simulink model "Complete_ballsegway_model"  (R2024b)
settings: Solver=VariableStepAuto  StartTime=0.0  StopTime=100  RelTol=1e-3
settings Model: Creator=sumit  LastModifiedBy=sumit

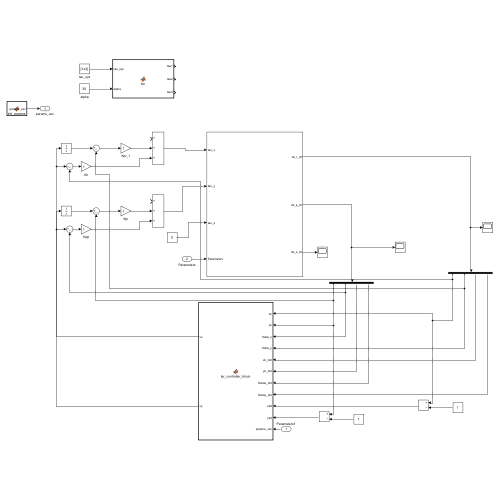
[thumbnail: Simulink's stored preview of the top-level diagram]
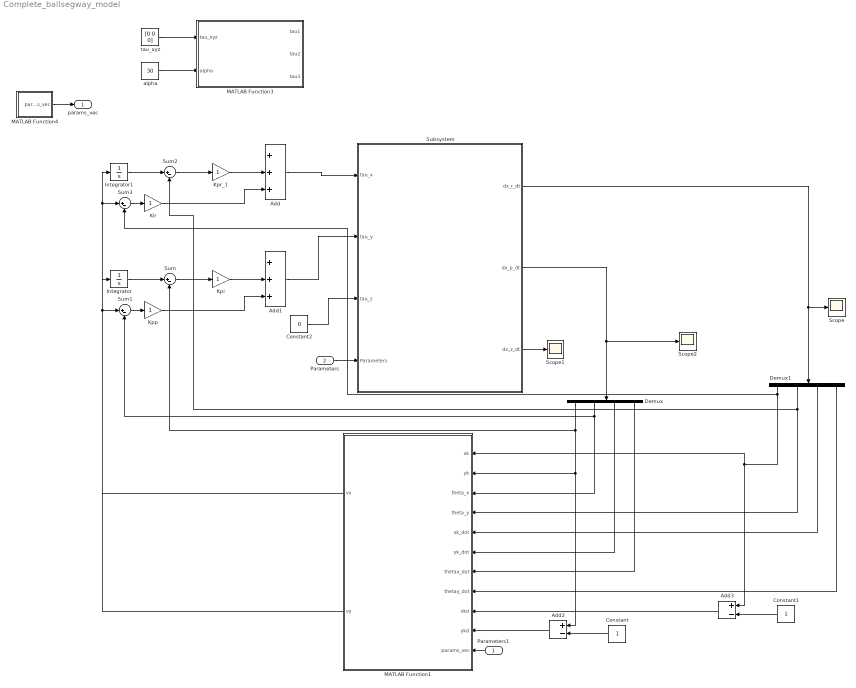
== system Complete_ballsegway_model ==
  Parameters1 : Inport
  Parameters : Inport  Port=2
  Add : Sum  Inputs=+++
  Add1 : Sum  Inputs=+++
  Add2 : Sum  Inputs=+-
  Add3 : Sum  Inputs=+-
  Constant : Constant
  Constant1 : Constant
  Constant2 : Constant  Value=0
  Demux : Demux
  Demux1 : Demux
  Integrator : Integrator
  Integrator1 : Integrator
  Kir : Gain
  Kpi : Gain
  Kpp : Gain
  Kpr_1 : Gain
  MATLAB Function1 : MATLAB Function  TreatAsAtomicUnit=on
  MATLAB Function3 : MATLAB Function  TreatAsAtomicUnit=on
  MATLAB Function4 : MATLAB Function  TreatAsAtomicUnit=on
  Scope : Scope
  Scope1 : Scope
  Scope2 : Scope
  Subsystem : Subsystem
  Sum{,1..3} (4 alike) : Sum  Inputs=|+-
  alpha : Constant  Value=30
  tau_xyz : Constant  Value=[0 0 0]
  params_vec : Outport
  wires:
  alpha/1 -> MATLAB Function3/2(alpha)
  tau_xyz/1 -> MATLAB Function3/1(tau_xyz)
  Subsystem/2(dx_p_dt) -> Demux/1, Scope2/1
  Subsystem/3(dx_z_dt) -> Scope1/1
  Add/1 -> Subsystem/1(tau_x)
  Add1/1 -> Subsystem/2(tau_y)
  Demux/1 -> Sum/2, Add2/1, MATLAB Function1/2(yk)
  Constant/1 -> Add2/2
  Kpi/1 -> Add1/2
  Sum/1 -> Kpi/1
  Integrator/1 -> Sum/1
  Add2/1 -> MATLAB Function1/10(ykd)
  Sum1/1 -> Kpp/1
  Kpp/1 -> Add1/3
  Demux/2 -> Sum1/2, MATLAB Function1/3(theta_x)
  Subsystem/1(dx_r_dt) -> Demux1/1, Scope/1
  MATLAB Function4/1(params_vec) -> params_vec/1
  Parameters/1 -> Subsystem/4(Parameters)
  MATLAB Function1/2(vy) -> Sum1/1, Integrator/1
  Demux/3 -> MATLAB Function1/6(yk_dot)
  Demux/4 -> MATLAB Function1/7(thetax_dot)
  Parameters1/1 -> MATLAB Function1/11(params_vec)
  Demux1/3 -> MATLAB Function1/5(xk_dot)
  Demux1/4 -> MATLAB Function1/8(thetay_dot)
  Constant1/1 -> Add3/2
  Add3/1 -> MATLAB Function1/9(xkd)
  Sum2/1 -> Kpr_1/1
  Kpr_1/1 -> Add/2
  Demux1/2 -> Sum2/2, MATLAB Function1/4(theta_y)
  Demux1/1 -> Sum3/2, Add3/1, MATLAB Function1/1(xk)
  Sum3/1 -> Kir/1
  MATLAB Function1/1(vx) -> Sum3/1, Integrator1/1
  Integrator1/1 -> Sum2/1
  Kir/1 -> Add/3
  Constant2/1 -> Subsystem/3(tau_z)

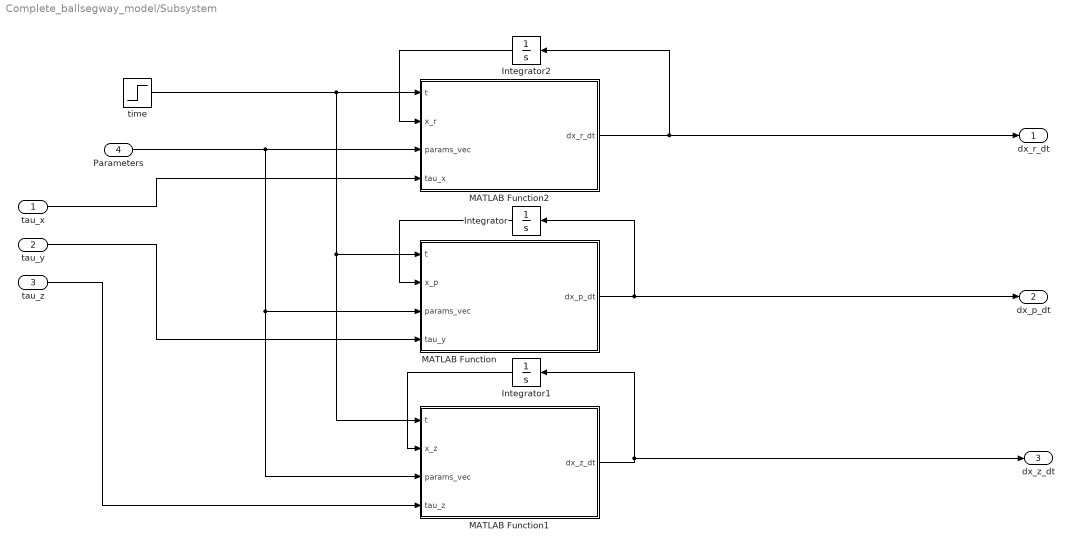
== system Complete_ballsegway_model/Subsystem ==
  tau_x : Inport
  tau_y : Inport  Port=2
  tau_z : Inport  Port=3
  Parameters : Inport  Port=4
  Integrator : Integrator  InitialCondition=[0; 0; 0; 0]
  Integrator1 : Integrator  InitialCondition=[0 ;0]
  Integrator2 : Integrator  InitialCondition=[0; 0; 0; 0]
  MATLAB Function : MATLAB Function  TreatAsAtomicUnit=on
  MATLAB Function1 : MATLAB Function  TreatAsAtomicUnit=on
  MATLAB Function2 : MATLAB Function  TreatAsAtomicUnit=on
  time : Step  After=10  SampleTime=0
  dx_r_dt : Outport
  dx_p_dt : Outport  Port=2
  dx_z_dt : Outport  Port=3
  wires:
  time/1 -> MATLAB Function1/1(t), MATLAB Function/1(t), MATLAB Function2/1(t)
  Integrator1/1 -> MATLAB Function1/2(x_z)
  Parameters/1 -> MATLAB Function/3(params_vec), MATLAB Function1/3(params_vec), MATLAB Function2/3(params_vec)
  Integrator2/1 -> MATLAB Function2/2(x_r)
  MATLAB Function1/1(dx_z_dt) -> Integrator1/1, dx_z_dt/1
  tau_z/1 -> MATLAB Function1/4(tau_z)
  Integrator/1 -> MATLAB Function/2(x_p)
  tau_y/1 -> MATLAB Function/4(tau_y)
  tau_x/1 -> MATLAB Function2/4(tau_x)
  MATLAB Function/1(dx_p_dt) -> Integrator/1, dx_p_dt/1
  MATLAB Function2/1(dx_r_dt) -> dx_r_dt/1, Integrator2/1

== matlab function Complete_ballsegway_model/Subsystem/MATLAB Function1 ==
  data: t input; dx_z_dt output; x_z input; params_vec input; tau_z input
function dx_z_dt = yaw_dynamics(t, x_z, params_vec, tau_z)
% yaw_dynamics.m
%
% 1-DOF yaw dynamic model for Ball Segway.
%
% State x_z = [theta_z ; theta_z_dot]
% params_vec = 20×1 numeric parameter vector (from init_params)
% Output dx_z_dt = state derivative (2×1)

%% ---------------------------------------------------------
% Unpack Parameters From Vector
%% ---------------------------------------------------------

mk  = params_vec(1);     %#ok<NASGU> (not used)
Ik  = params_vec(2);
ma  = params_vec(3);     %#ok<NASGU>
Ix  = params_vec(4);     %#ok<NASGU>
Iy  = params_vec(5);
Iz  = params_vec(6);
l   = params_vec(7);     %#ok<NASGU>
alpha_rad = params_vec(8);
rk  = params_vec(9);
rw  = params_vec(10);
bx  = params_vec(11);    %#ok<NASGU>
dx  = params_vec(12);    %#ok<NASGU>
by  = params_vec(13);    %#ok<NASGU>
dy  = params_vec(14);    %#ok<NASGU>
bry = params_vec(15);    %#ok<NASGU>
dry = params_vec(16);    %#ok<NASGU>
brx = params_vec(17);    %#ok<NASGU>
drx = params_vec(18);    %#ok<NASGU>
g   = params_vec(19);    %#ok<NASGU>
k_motor = params_vec(20); %#ok<NASGU>

% Keep notation same as your original code
I_k_param = Ik;
I_w = Iy;


%% ---------------------------------------------------------
% Extract States
%% ---------------------------------------------------------

theta_z     = x_z(1);
theta_z_dot = x_z(2);


%% ---------------------------------------------------------
% Yaw Dynamics (Eq. 13)
%% ---------------------------------------------------------

num = I_k_param * (rk / rw) * tau_z;

den = I_k_param * Iz + ...
      3 * (I_k_param + Iz) * I_w * (rk / rw)^2 * sin(alpha_rad)^2;

theta_z_ddot = num / den;


%% ---------------------------------------------------------
% Return Derivative
%% ---------------------------------------------------------

dx_z_dt = [ theta_z_dot ;
            theta_z_ddot ];

end

== matlab function Complete_ballsegway_model/Subsystem/MATLAB Function ==
  data: t input; dx_p_dt output; x_p input; params_vec input; tau_y input
function dx_p_dt = pitch_dynamics(t, x_p, params_vec, tau_y)
% pitch_dynamics.m
%
% 2-DOF dynamic model in the X–Z plane (pitch plane).
%
% State x_p = [x_k ; theta_y ; x_k_dot ; theta_y_dot]
% params_vec = 20×1 vector from init_params()
% Output dx_p_dt = state derivative (4×1)

%% ---------------------------------------------------------
% Unpack Parameters from Vector
%% ---------------------------------------------------------

mk  = params_vec(1);     % ball mass
Ik  = params_vec(2);     % ball inertia
ma  = params_vec(3);     % body mass
Ix  = params_vec(4);     % inertia about x
Iy  = params_vec(5);     % inertia about y
Iz  = params_vec(6);     % inertia about z
l   = params_vec(7);     % COM height
alpha_rad = params_vec(8); % zenith angle
rk  = params_vec(9);     % ball radius
rw  = params_vec(10);    % omniwheel radius
bx  = params_vec(11);
dx  = params_vec(12);
by  = params_vec(13);
dy  = params_vec(14);
bry = params_vec(15);
dry = params_vec(16);
brx = params_vec(17);
drx = params_vec(18);
g   = params_vec(19);    % gravity
k_motor = params_vec(20);

% Keep original notation
I_k_param = Ik;
I_w = Iy;    % consistent with roll dynamics formulation


%% ---------------------------------------------------------
% Extract State Variables
%% ---------------------------------------------------------

x_k         = x_p(1);
theta_y     = x_p(2);
x_k_dot     = x_p(3);
theta_y_dot = x_p(4);

q_y_dot = [x_k_dot ; theta_y_dot];


%% ---------------------------------------------------------
% Mass Matrix M(q)   (Eq. 8)
%% ---------------------------------------------------------

M11 = mk + (I_k_param / rk^2) + ma + ...
      (3*I_w*cos(alpha_rad)^2) / (2*rw^2);

M12 =   ma*l*cos(theta_y) ...
      - (3*I_w*cos(alpha_rad)^2)/(2*rw^2) * rk;

M21 = M12;

M22 = ma*l^2 + ...
      (3*I_w*rk^2*cos(alpha_rad)^2)/(2*rw^2) + Iy;

M_y = [M11 M12; M21 M22];


%% ---------------------------------------------------------
% Coriolis–Centrifugal Vector
%% ---------------------------------------------------------

C_y = [ 0                            -ma*l*theta_y_dot*sin(theta_y);
        0                             0 ];


%% ---------------------------------------------------------
% Gravity Vector
%% ---------------------------------------------------------

G_y = [0;
       -ma*g*l*sin(theta_y)];


%% ---------------------------------------------------------
% Friction Vector (ignored)
%% ---------------------------------------------------------

D_y = [0; 0];


%% ---------------------------------------------------------
% Input Torque Vector
%% ---------------------------------------------------------

Q_y = [ -(1/rw) * tau_y ;
         (rk/rw) * tau_y ];


%% ---------------------------------------------------------
% Solve q¨ = M⁻¹ (Q – C q̇ – D – G)
%% ---------------------------------------------------------

q_y_ddot = M_y \ (Q_y - C_y*q_y_dot - D_y - G_y);


%% ---------------------------------------------------------
% Output State Derivatives
%% ---------------------------------------------------------

dx_p_dt = [ x_k_dot ;
            theta_y_dot ;
            q_y_ddot(1) ;
            q_y_ddot(2) ];

end

== matlab function Complete_ballsegway_model/Subsystem/MATLAB Function2 ==
  data: t input; dx_r_dt output; x_r input; params_vec input; tau_x input
function dx_r_dt = roll_dynamics(t, x_r, params_vec, tau_x)
% roll_dynamics.m
%
% State vector x_r = [y_k, theta_x, y_k_dot, theta_x_dot]'

%% 1. Unpack State
y_k         = x_r(1);
theta_x     = x_r(2);
y_k_dot     = x_r(3);
theta_x_dot = x_r(4);
q_x_dot     = [y_k_dot; theta_x_dot];

%% 2. Unpack parameters from vector
mk  = params_vec(1);
Ik  = params_vec(2);
ma  = params_vec(3);
Ix  = params_vec(4);
Iy  = params_vec(5);
Iz  = params_vec(6);
l   = params_vec(7);
alpha_rad = params_vec(8);
rk  = params_vec(9);
rw  = params_vec(10);
bx  = params_vec(11);
dx  = params_vec(12);
by  = params_vec(13);   % USED
dy  = params_vec(14);   % USED
bry = params_vec(15);
dry = params_vec(16);
brx = params_vec(17);   % USED
drx = params_vec(18);   % USED
g   = params_vec(19);
k_motor = params_vec(20);

%% 3. Dynamics Matrices

% Mass Matrix
M11 = mk + (Ik / rk^2) + ma + (3*Iy*cos(alpha_rad)^2)/(2*rw^2);
M12 = (3*Iy*cos(alpha_rad)^2)/(2*rw^2)*rk - ma*l*cos(theta_x);
M21 = M12;
M22 = ma*l^2 + (3*Iy*rk^2*cos(alpha_rad)^2)/(2*rw^2) + Ix;
M_x = [M11 M12; M21 M22];

% Coriolis Matrix
C_x = [ 0                     ma*l*theta_x_dot*sin(theta_x);
        0                     0 ];

% Gravity Vector
G_x = [ 0 ;
       -ma*g*l*sin(theta_x) ];

%% 4. Friction / Damping Vector (NEW)
% D(q̇) = [by*y_k_dot + dy*sign(y_k_dot) ;
%         brx*theta_x_dot + drx*sign(theta_x_dot)]

D1 = by * y_k_dot     + dy  * sign(y_k_dot);
D2 = brx * theta_x_dot + drx * sign(theta_x_dot);
D_x = [D1 ; D2];

%% 5. Control torque vector
Q_x = [ (1/rw)*tau_x ;
         (rk/rw)*tau_x ];

%% 6. Compute accelerations
q_x_ddot = M_x \ (Q_x - C_x*q_x_dot - D_x - G_x);

%% 7. Output derivative
dx_r_dt = [
    y_k_dot ;
    theta_x_dot ;
    q_x_ddot(1) ;
    q_x_ddot(2)
];

end

== matlab function Complete_ballsegway_model/MATLAB Function3 ==
  data: tau_xyz input; tau1 output; alpha input; tau2 output; tau3 output
function [tau1, tau2, tau3] = fcn(tau_xyz, alpha)
% Converts global torques [tau_x; tau_y; tau_z]
% into individual wheel torques tau1, tau2, tau3
%
% EXACT equation provided in the image.

%% Precompute trig values
c_alpha = cos(alpha);
s_alpha = sin(alpha);
sqrt3 = sqrt(3);

% Avoid division by zero
if abs(c_alpha) < eps
    c_alpha = eps * sign(c_alpha + (c_alpha==0));
end
if abs(s_alpha) < eps
    s_alpha = eps * sign(s_alpha + (s_alpha==0));
end

%% Matrix M (exact from your equation)
M = [  2/(3*c_alpha),              0,               1/(3*s_alpha);
      -1/(3*c_alpha),   sqrt3/(3*c_alpha),         1/(3*s_alpha);
      -1/(3*c_alpha),  -sqrt3/(3*c_alpha),         1/(3*s_alpha) ];

%% Compute wheel torques
tau_vec = M * tau_xyz(:);

%% Output individually
tau1 = tau_vec(1);
tau2 = tau_vec(2);
tau3 = tau_vec(3);

end

== matlab function Complete_ballsegway_model/MATLAB Function4 ==
  data: params_vec output
function params_vec = init_params()
% init_params.m
% Returns parameters as a 20×1 vector (NO STRUCT)

mk  = 19.6;                   % (1) ball mass
Ik  = 0.38;                   % (2) ball inertia
ma  = 68;                     % (3) body mass
Ix  = 12.1;                   % (4) body inertia x
Iy  = 11.67;                  % (5) body inertia y
Iz  = 1.08;                   % (6) body inertia z
l   = 0.38;                   % (7) COM height
a   = deg2rad(65.5);          % (8) zenith angle
rk  = 0.22;                   % (9) ball radius
rw  = 0.10;                   % (10) omniwheel radius
bx  = 0.10;                   % (11) viscous friction xz
dx  = 0.01;                   % (12) coulomb friction xz
by  = 0.10;                   % (13) viscous friction yz
dy  = 0.01;                   % (14) coulomb friction yz
bry = 0.12;                   % (15) body/ball viscous xz
dry = 0.02;                   % (16) coulomb xz
brx = 0.12;                   % (17) body/ball viscous yz
drx = 0.02;                   % (18) coulomb yz
g   = 9.81;                   % (19) gravity
k_motor = 1;                  % (20) motor constant

% Return as vector
params_vec = [
    mk; Ik; ma; Ix; Iy; Iz;
    l; a; rk; rw;
    bx; dx; by; dy;
    bry; dry; brx; drx;
    g; k_motor
];
end

== matlab function Complete_ballsegway_model/MATLAB Function1 ==
  data: vx output; xk input; yk input; theta_x input; theta_y input; xk_dot input; yk_dot input; thetax_dot input; thetay_dot input; xkd input; ykd input; params_vec input; vy output
function [vx, vy] = lqr_controller_block(xk, yk, theta_x, theta_y, xk_dot, yk_dot, thetax_dot, thetay_dot, xkd, ykd, params_vec)
% LQR controller with parameter input
% Inputs: system state, desired pos, and parameter vector (length = 20)
% Outputs: vx, vy — reference ball velocities

% Unpack parameters
mk  = params_vec(1);
Ik  = params_vec(2);
ma  = params_vec(3);
Ix  = params_vec(4);
Iy  = params_vec(5);
Iz  = params_vec(6);
l   = params_vec(7);
a   = params_vec(8);
rk  = params_vec(9);
rw  = params_vec(10);
bx  = params_vec(11);
dx  = params_vec(12);
by  = params_vec(13);
dy  = params_vec(14);
bry = params_vec(15);
dry = params_vec(16);
brx = params_vec(17);
drx = params_vec(18);
g   = params_vec(19);
k_m = params_vec(20);

% Common term
mau  = (2*rw*l*(Ix + ma*l^2) + 3*l*(ma+mk)*rk^3*cos(a)^2 + ...
        2*l*(ma+mk)*rk^2 + 3*(l*(Ix + 2*ma*l))*rw^2*cos(a)^2 + ...
        2*ma*mk*l^2*rw^2*cos(a)^2);

maup = (2*rw*l*(Iy + ma*l^2) + 3*l*(ma+mk)*rk^3*cos(a)^2 + ...
        2*l*(ma+mk)*rk^2 + 3*(l*(Iy + 2*ma*l))*rk^2*cos(a)^2 + ...
        2*ma*mk*l^2*rk^2*cos(a)^2);

% Roll A_r and B_r
Ar = zeros(5,5);
Br = zeros(5,2);

Ar(1,3) = 1;
Ar(2,4) = 1;
Ar(3,1) = -k_m*rk*rw*(ma*l^2 + ma*l + l)/mau;
Ar(3,3) = -brx/mau;
Ar(3,4) = -drx/mau;
Ar(3,5) = k_m*rk*rw*(ma*l^2 + ma*l + l)/mau;
Br(3,1) = 2*k_m*rk*rw*(ma*l^2 + l)/mau;
Br(3,2) = 2*k_m*rk*rw*(l + ma*l)/mau;

% Pitch A_p and B_p
Ap = zeros(5,5);
Bp = zeros(5,2);

Ap(1,3) = 1;
Ap(2,4) = 1;
Ap(3,1) = k_m*rk*rw*(ma*l^2 + ma*l + l)/maup;
Ap(3,3) = -bry/maup;
Ap(3,4) = -dry/maup;
Ap(3,5) = k_m*rk*rw*(ma*l^2 + ma*l + l)/maup;
Bp(3,1) = 2*k_m*rk*rw*(ma*l^2 + l)/maup;
Bp(3,2) = 2*k_m*rk*rw*(l + ma*l)/maup;

% Augment A and B (add integrator state)
Cpos = [1 0 0 0 0];

Aroll_aug = [Ar, zeros(5,1); -Cpos, 0];
Broll_aug = [Br; 0 0];

Apitch_aug = [Ap, zeros(5,1); -Cpos, 0];
Bpitch_aug = [Bp; 0 0];

% Define Q and R (tunable)
Q = diag([10 200 1 50 200 20]);  % x, θ, ẋ, θ̇, x5
R = 0.5 * eye(2);

% Solve LQR
[Kroll,~,~] = lqr(Aroll_aug, Broll_aug, Q, R);
[Kpitch,~,~] = lqr(Apitch_aug, Bpitch_aug, Q, R);

% Build augmented states
persistent int_x int_y
if isempty(int_x)
    int_x = 0;
    int_y = 0;
end

% Integrate errors (Euler approx)
Ts = 0.001; % sampling time
int_x = int_x + (xkd - xk)*Ts;
int_y = int_y + (ykd - yk)*Ts;

x_ra = [xk; theta_x; xk_dot; thetax_dot; int_x];
x_pa = [yk; theta_y; yk_dot; thetay_dot; int_y];

% LQR output: reference ball velocities
vx = -Kroll * x_ra;
vy = -Kpitch * x_pa;

end
